simulink model "chlnet"  (Simulink 10.0)
settings: Solver=ode45  StartTime=1  StopTime=length(t)  RelTol=1e-3  EnableMultiTasking=on
undefined symbols (not defined in the file): maxdata, mindata
libraries: ann x1, simulink3 x1
settings Model: Creator=Giampy  LastModifiedBy=bhisma  ExtModeTrigMode=oneshot  ExtModeArmWhenConnect=off
settings DataIOCC: Decimation=35*50  SignalLoggingSaveFormat=ModelDataLogs  SaveOutput=off  SaveTime=off  OutputTimes=[0:50:3900]
settings OptimizationCC: BlockReduction=off  BooleanDataType=off  InitFltsAndDblsToZero=on  LifeSpan=auto
settings DebuggingCC: SaveWithParameterizedLinksMsg=none  SignalResolutionControl=TryResolveAllWithWarning  MultiTaskDSMMsg=warning  MultiTaskCondExecSysMsg=none  SFUnexpectedBacktrackingDiag=error  SFNoUnconditionalDefaultTransitionDiag=error  SFExecutionAtInitializationDiag=warning  ArithmeticOperatorsInVariantConditions=error
settings HardwareCC: ProdBitPerPointer=64  ProdBitPerSizeT=64  ProdBitPerPtrDiffT=64  ProdLargestAtomicFloat=Float  ProdIntDivRoundTo=Zero  ProdEndianess=LittleEndian  ProdWordSize=64  ProdHWDeviceType=Intel->x86-64 (Windows64)  TargetUnknown=on
settings SFSimCC: SimUseLocalCustomCode=on  CustomCodeUndefinedFunction=FilterOut
settings RTWCC: RTWUseLocalCustomCode=on
settings CodeAppCC: StateflowObjectComments=off
settings GRTTargetCC: TargetFcnLib=ansi_tfl_tmw.mat
settings ConfigComp: CovMetricSettings=dwe  CovHtmlReporting=off  CovSaveCumulativeToWorkspaceVar=off  CovSaveSingleToWorkspaceVar=off

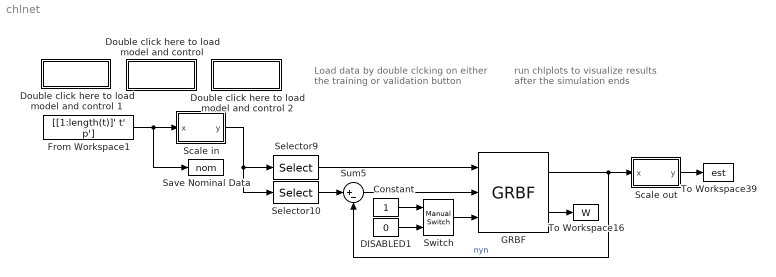
== system chlnet ==
  note: run chlplots to visualize results
      | after the simulation ends
  note: Load data by double clcking on either
      | the training or validation button
  Constant : Constant
  DISABLED1 : Constant  Value=0
  "Double click here to load model and control " : Subsystem
      settings: OpenFcn=load choles_all;t=t(:,1:130);p=p(:,1:130);mindata=min([t' p']);maxdata=max([t' p']);W=zeros(1,((21+2)*100+2)*3);
      mask Display: disp('Training\nData')
  Double click here to load model and control 1 : Subsystem
      settings: OpenFcn=edit('training.txt')
      mask Display: disp('Readme')
  Double click here to load model and control 2 : Subsystem
      settings: OpenFcn=load choles_all; t=t(:,131:end);p=p(:,131:end); load chl_W
      mask Display: disp('Validation\nData')
  From Workspace1 : FromWorkspace  VariableName=[[1:length(t)]' t' p']  SampleTime=1
  GRBF : ann/GRBF  dim=[21 3]  nwrap="[100   0.4         1e10           1]"  eta=[0.0001 0.0001 0.0001]  gam=[1e-6 1e-6 1e-6]*0  lim=[1e9 1e9 1e9]  e1=0.1  e2="[0.6  0.6  1]"  e3=[0.02 0.5]  x0=W(end,:) % zeros(((21+2)*100+2)*3,1) %  T=1
  Save Nominal Data : ToWorkspace  VariableName=nom  SampleTime=1
  Scale in : Subsystem  mask(Scale){xmin=mindata, xmax=maxdata, ymin=-ones(size(mindata)), ymax=ones(size(maxdata))}
      mask prompts: xmin "x min"; xmax "x max"; ymin "y min"; ymax "y max"
      mask help:
      | Scales the input vector x, ranging from xmin to xmax,
      |    to an output vector y, ranging from ymin to ymax
      mask Help:
      | Scales the input vector x, ranging from xmin to xmax,
      |    to an output vector y, ranging from ymin to ymax
  Scale out : Subsystem  mask(Scale){xmin=-ones(1,3), xmax=ones(1,3), ymin=mindata(1:3), ymax=maxdata(1:3)}
      mask prompts: xmin "x min"; xmax "x max"; ymin "y min"; ymax "y max"
      mask help:
      | Scales the input vector x, ranging from xmin to xmax,
      |    to an output vector y, ranging from ymin to ymax
      mask Help:
      | Scales the input vector x, ranging from xmin to xmax,
      |    to an output vector y, ranging from ymin to ymax
  Selector10 : Selector  InputPortWidth=24  IndexOptions=Index vector (dialog)  Indices=1:3  OutputSizes=1
  Selector9 : Selector  InputPortWidth=24  IndexOptions=Index vector (dialog)  Indices=4:24  OutputSizes=1
  Sum5 : Sum  Inputs=|+-  SaturateOnIntegerOverflow=on  InputSameDT=on  OutDataTypeStr=Inherit: Same as first input
  Switch : simulink3/Nonlinear/Manual Switch  sw=1  action=0
      settings: SourceProductName=Simulink  SourceProductBaseCode=SL
  To Workspace16 : ToWorkspace  VariableName=W  SampleTime=1
  To Workspace39 : ToWorkspace  VariableName=est  SampleTime=1
  wires:
  From Workspace1/1 -> Save Nominal Data/1, Scale in/1(x)
  Scale in/1(y) -> Selector9/1, Selector10/1
  Selector10/1 -> Sum5/1
  Selector9/1 -> GRBF/1
  Scale out/1(y) -> To Workspace39/1
  GRBF/1 -> Sum5/2, Scale out/1(x)  "nyn"
  GRBF/2 -> To Workspace16/1
  Constant/1 -> Switch/1
  DISABLED1/1 -> Switch/2
  Sum5/1 -> GRBF/2
  Switch/1 -> GRBF/3

== system chlnet/Double click here to load model and control  ==

== system chlnet/Double click here to load model and control 1 ==

== system chlnet/Double click here to load model and control 2 ==

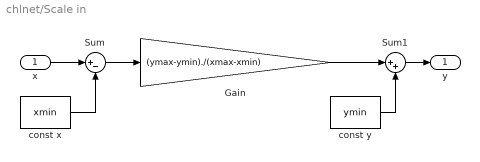
== system chlnet/Scale in ==
  x : Inport
  Gain : Gain  Gain=(ymax-ymin)./(xmax-xmin)  SaturateOnIntegerOverflow=on  OutDataTypeStr=Inherit: Same as input  ParamDataTypeStr=Inherit: Same as input
  Sum : Sum  Inputs=|+-  SaturateOnIntegerOverflow=on  InputSameDT=on  OutDataTypeStr=Inherit: Same as first input
  Sum1 : Sum  Inputs=|++  SaturateOnIntegerOverflow=on  InputSameDT=on  OutDataTypeStr=Inherit: Same as first input
  const x : Constant  Value=xmin
  const y : Constant  Value=ymin
  y : Outport
  wires:
  x/1 -> Sum/1
  Sum/1 -> Gain/1
  const x/1 -> Sum/2
  Gain/1 -> Sum1/1
  Sum1/1 -> y/1
  const y/1 -> Sum1/2

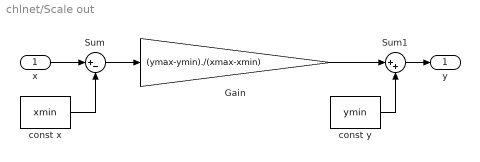
== system chlnet/Scale out ==
  x : Inport
  Gain : Gain  Gain=(ymax-ymin)./(xmax-xmin)  SaturateOnIntegerOverflow=on  OutDataTypeStr=Inherit: Same as input  ParamDataTypeStr=Inherit: Same as input
  Sum : Sum  Inputs=|+-  SaturateOnIntegerOverflow=on  InputSameDT=on  OutDataTypeStr=Inherit: Same as first input
  Sum1 : Sum  Inputs=|++  SaturateOnIntegerOverflow=on  InputSameDT=on  OutDataTypeStr=Inherit: Same as first input
  const x : Constant  Value=xmin
  const y : Constant  Value=ymin
  y : Outport
  wires:
  const y/1 -> Sum1/2
  Sum1/1 -> y/1
  Gain/1 -> Sum1/1
  const x/1 -> Sum/2
  Sum/1 -> Gain/1
  x/1 -> Sum/1
